simulink model "sampleModel1607_5"  (R2023a)
settings: Solver=VariableStepAuto  StartTime=0.0  StopTime=10.0  RelTol=1e-3
libraries: hdlsllib x2, simulink x1
settings Model: Creator=user1  LastModifiedBy=user1

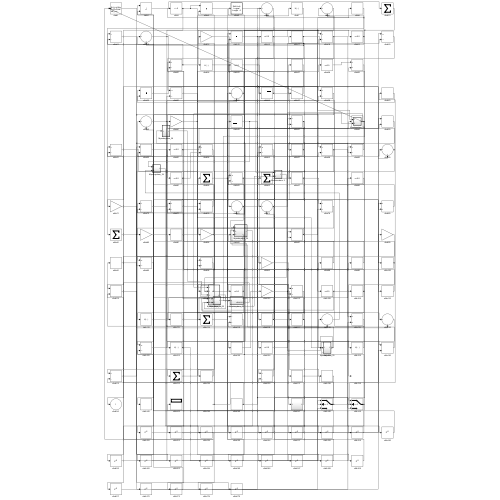
[thumbnail: Simulink's stored preview of the top-level diagram]
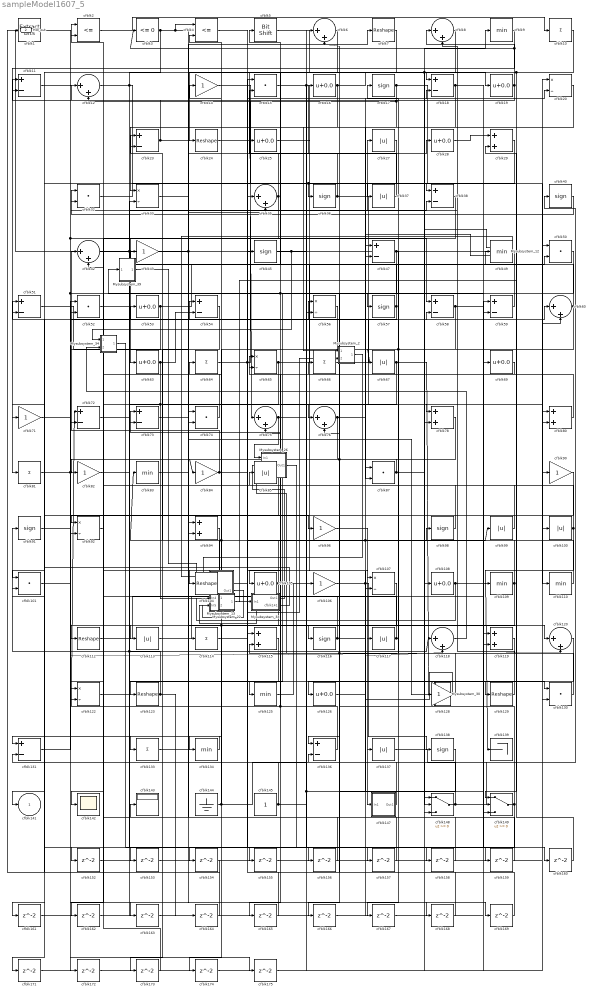
== system sampleModel1607_5 ==
  Mysubsystem_12 : Subsystem  TreatAsAtomicUnit=on  RTWFcnName=Mysubsystem_12
      settings: RTWFcnNameOpts=User specified  RTWFileNameOpts=Use function name
  Mysubsystem_13 : Subsystem  TreatAsAtomicUnit=on  RTWFcnName=Mysubsystem_13
      settings: RTWFcnNameOpts=User specified  RTWFileNameOpts=Use function name
  Mysubsystem_2 : Subsystem  TreatAsAtomicUnit=on  RTWFcnName=Mysubsystem_2
      settings: RTWFcnNameOpts=User specified  RTWFileNameOpts=Use function name
  Mysubsystem_22 : Subsystem  TreatAsAtomicUnit=on  RTWFcnName=Mysubsystem_22
      settings: RTWFcnNameOpts=User specified  RTWFileNameOpts=Use function name
  Mysubsystem_26 : Subsystem  TreatAsAtomicUnit=on  RTWFcnName=Mysubsystem_26
      settings: RTWFcnNameOpts=User specified  RTWFileNameOpts=Use function name
  Mysubsystem_30 : Subsystem  TreatAsAtomicUnit=on  RTWFcnName=Mysubsystem_30
      settings: RTWFcnNameOpts=User specified  RTWFileNameOpts=Use function name
  Mysubsystem_33 : Subsystem  TreatAsAtomicUnit=on  RTWFcnName=Mysubsystem_33
      settings: RTWFcnNameOpts=User specified  RTWFileNameOpts=Use function name
  Mysubsystem_34 : Subsystem  TreatAsAtomicUnit=on  RTWFcnName=Mysubsystem_34
      settings: RTWFcnNameOpts=User specified  RTWFileNameOpts=Use function name
  Mysubsystem_39 : Subsystem  TreatAsAtomicUnit=on  RTWFcnName=Mysubsystem_39
      settings: RTWFcnNameOpts=User specified  RTWFileNameOpts=Use function name
  cfblk1 : simulink/Logic and Bit Operations/Extract Bits  bitsToExtract=Upper half  numBits=8  bitIdxRange=[0 7]  outScalingMode=Preserve fixed-point scaling
      settings: LibrarySourceBlock=|
      | hdlsllib/Logic and Bit
      | Operations/Extract Bits
  cfblk{10,64,66,81,114,133} (6 alike) : Sum  Inputs=+  OutDataTypeStr=uint8
  cfblk{27,37,67,85,99..100,113,117,137} (9 alike) : Abs  OutDataTypeStr=uint8  SaturateOnIntegerOverflow=off
  cfblk{15,32,50,52,74,87,101,130} (8 alike) : DotProduct  OutDataTypeStr=uint8
  cfblk{7,24,104,112,123,129} (6 alike) : Reshape
  cfblk{16,19,25,28,53,63,69,105,108,126} (10 alike) : Bias  Bias=0.0  SaturateOnIntegerOverflow=off
  cfblk{14,43,71,82,84,90,96,106,128} (9 alike) : Gain  OutDataTypeStr=uint8
  cfblk{20,33,56,65,92,107,122} (7 alike) : Product  Inputs=*/  OutDataTypeStr=uint8  RndMeth=Zero  SaturateOnIntegerOverflow=on
  cfblk{9,49,83,109..110,125,134} (7 alike) : MinMax  OutDataTypeStr=uint8
  cfblk{11,18,23,38,47,51,54,58..59,72..73,131,136} (13 alike) : Sum  Inputs=+-  OutDataTypeStr=uint8
  cfblk{29,78,80,94,115,119} (6 alike) : Sum  OutDataTypeStr=uint8
  cfblk{17,36,40,45,57,91,98,116,138} (9 alike) : Signum
  cfblk{6,8,12,35,42,60,75..76,118,120} (10 alike) : Sum  Inputs=|++  OutDataTypeStr=uint8
  cfblk139 : Terminator
  cfblk142 : Scope
  cfblk143 : Display
  cfblk144 : Ground
  cfblk145 : Constant  OutDataTypeStr=uint8  SampleTime=-1
  cfblk147 : Subsystem
      settings: LibrarySourceBlock=|
      | hdlsllib/Ports &
      | Subsystems/Subsystem
  cfblk148 : Switch  OutDataTypeStr=uint8  SaturateOnIntegerOverflow=off  InputSameDT=off
  cfblk149 : Switch  OutDataTypeStr=uint8  SaturateOnIntegerOverflow=off  InputSameDT=off
  cfblk{152..169,171..175} (23 alike) : Delay  SampleTime=1
  cfblk2 : RelationalOperator  Operator=<=  OutDataTypeStr=boolean  InputSameDT=off
  cfblk3 : hdlsllib/Logic and Bit Operations/Compare To Zero  relop=<=  OutDataTypeStr=uint8
  cfblk4 : RelationalOperator  Operator=<=  OutDataTypeStr=boolean  InputSameDT=off
  cfblk5 : hdlsllib/Logic and Bit Operations/Bit Shift  mode=Shift Left Logical  N=0
  cfblk141 : Outport  OutDataTypeStr=uint8  VectorParamsAs1DForOutWhenUnconnected=off
  Hdl_out : Outport  Port=2  OutDataTypeStr=uint8
  wires:
  cfblk10/1 -> Mysubsystem_12/1(In1), cfblk75/1, cfblk149/1
  cfblk27/1 -> cfblk73/1
  cfblk9/1 -> cfblk81/1
  cfblk47/1 -> cfblk67/1, cfblk167/1, cfblk123/1
  cfblk64/1 -> cfblk27/1, cfblk107/1
  cfblk35/1 -> cfblk63/1, cfblk15/2
  cfblk6/1 -> Mysubsystem_39/1(In1), cfblk165/1
  cfblk75/1 -> Mysubsystem_26/1(In1), cfblk129/1
  cfblk84/1 -> cfblk42/1, cfblk18/2
  cfblk2/1 -> cfblk10/1
  cfblk136/1 -> cfblk72/1, cfblk85/1
  cfblk120/1 -> cfblk143/1
  cfblk78/1 -> cfblk84/1, cfblk116/1
  cfblk108/1 -> Mysubsystem_13/4(In4), cfblk139/1
  cfblk110/1 -> cfblk83/1, cfblk54/1
  cfblk24/1 -> cfblk100/1
  cfblk125/1 -> cfblk106/1
  cfblk32/1 -> cfblk38/1
  cfblk67/1 -> cfblk128/1, cfblk125/1
  cfblk15/1 -> cfblk147/1(In1), cfblk107/2
  cfblk99/1 -> cfblk65/1
  cfblk3/1 -> cfblk4/1, cfblk120/1, cfblk71/1
  cfblk60/1 -> cfblk126/1, cfblk23/1
  cfblk107/1 -> cfblk133/1, cfblk174/1
  cfblk65/1 -> cfblk49/1, cfblk113/1
  cfblk137/1 -> cfblk40/1
  cfblk149/1 -> cfblk66/1, cfblk171/1
  cfblk96/1 -> cfblk137/1
  cfblk106/1 -> cfblk138/1, cfblk118/2
  cfblk123/1 -> cfblk91/1, cfblk164/1
  cfblk36/1 -> cfblk110/1, cfblk25/1
  cfblk117/1 -> cfblk4/2, cfblk157/1
  cfblk130/1 -> cfblk17/1
  cfblk57/1 -> cfblk5/1, cfblk51/2
  cfblk109/1 -> cfblk43/1, cfblk162/1
  cfblk104/1 -> cfblk73/2, cfblk98/1
  cfblk82/1 -> cfblk56/1
  cfblk49/1 -> Mysubsystem_33/1(In1), cfblk117/1
  cfblk20/1 -> cfblk105/1
  cfblk98/1 -> cfblk2/1
  cfblk94/1 -> cfblk112/1
  cfblk8/1 -> cfblk24/1
  cfblk134/1 -> cfblk131/1
  cfblk129/1 -> cfblk32/1
  cfblk105/1 -> cfblk14/1, cfblk173/1
  cfblk119/1 -> cfblk115/2
  cfblk17/1 -> cfblk33/1, cfblk12/2, cfblk60/2
  cfblk37/1 -> cfblk16/1
  cfblk38/1 -> cfblk142/1
  cfblk7/1 -> cfblk75/2
  cfblk14/1 -> cfblk37/1
  cfblk126/1 -> cfblk99/1, cfblk20/2
  cfblk76/1 -> Mysubsystem_12/2(In2), cfblk94/2
  cfblk128/1 -> Mysubsystem_26/3(In3), cfblk6/2
  cfblk28/1 -> cfblk29/1
  cfblk42/1 -> cfblk38/2, cfblk130/1
  cfblk116/1 -> cfblk2/2, cfblk149/3
  cfblk18/1 -> cfblk119/1, cfblk87/2
  cfblk19/1 -> cfblk8/1, cfblk3/1, cfblk11/2
  cfblk63/1 -> Mysubsystem_22/1(In1), cfblk92/1, cfblk54/2
  cfblk5/1 -> cfblk148/2
  cfblk59/1 -> cfblk57/1
  cfblk80/1 -> cfblk8/2
  cfblk100/1 -> cfblk109/1, cfblk23/2
  cfblk16/1 -> Mysubsystem_2/1(In1), cfblk19/1
  cfblk72/1 -> cfblk78/1
  cfblk56/1 -> cfblk104/1
  cfblk33/1 -> cfblk35/2
  cfblk25/1 -> cfblk58/1
  cfblk144/1 -> cfblk64/1, cfblk6/1
  cfblk147/1(Out1) -> cfblk51/1
  cfblk45/1 -> Mysubsystem_34/1(In1), cfblk159/1
  cfblk131/1 -> cfblk52/1
  cfblk90/1 -> cfblk122/1
  cfblk51/1 -> cfblk74/2
  cfblk87/1 -> cfblk82/1, cfblk9/1
  cfblk122/1 -> cfblk50/2, cfblk118/1
  cfblk1/1 -> cfblk59/2, cfblk120/2
  cfblk12/1 -> cfblk108/1, cfblk18/1, cfblk154/1
  cfblk113/1 -> cfblk45/1
  cfblk69/1 -> cfblk65/2
  cfblk85/1 -> cfblk101/1
  cfblk74/1 -> cfblk12/1
  cfblk58/1 -> cfblk76/1, cfblk160/1
  cfblk53/1 -> cfblk20/1, cfblk92/2
  cfblk50/1 -> cfblk136/1
  cfblk23/1 -> cfblk11/1, cfblk169/1
  cfblk11/1 -> cfblk47/2, cfblk168/1
  cfblk112/1 -> cfblk69/1
  cfblk83/1 -> cfblk7/1
  cfblk115/1 -> cfblk134/1
  cfblk66/1 -> cfblk58/2
  cfblk81/1 -> cfblk53/1, cfblk96/1
  cfblk52/1 -> cfblk80/2
  cfblk148/1 -> cfblk90/1, cfblk52/2
  cfblk133/1 -> cfblk94/1
  cfblk29/1 -> cfblk36/1, cfblk161/1
  cfblk43/1 -> cfblk114/1, cfblk28/1
  cfblk40/1 -> cfblk32/2
  cfblk145/1 -> cfblk60/1, cfblk149/2, cfblk101/2
  cfblk92/1 -> cfblk152/1
  cfblk152/1 -> cfblk35/1
  cfblk54/1 -> cfblk153/1
  cfblk153/1 -> cfblk50/1
  cfblk154/1 -> cfblk1/1
  cfblk155/1 -> cfblk80/1
  cfblk4/1 -> cfblk156/1
  cfblk156/1 -> cfblk42/2
  cfblk157/1 -> cfblk122/2
  cfblk158/1 -> cfblk74/1
  cfblk159/1 -> cfblk76/2
  cfblk160/1 -> cfblk29/2
  cfblk161/1 -> cfblk78/2
  cfblk162/1 -> cfblk33/2
  cfblk91/1 -> cfblk163/1
  cfblk163/1 -> cfblk119/2
  cfblk164/1 -> cfblk131/2
  cfblk165/1 -> cfblk115/1
  cfblk138/1 -> cfblk166/1
  cfblk166/1 -> cfblk47/1
  cfblk167/1 -> cfblk148/3
  cfblk168/1 -> cfblk15/1
  cfblk169/1 -> cfblk136/2
  cfblk171/1 -> cfblk56/2
  cfblk71/1 -> cfblk172/1
  cfblk172/1 -> cfblk59/1
  cfblk173/1 -> cfblk72/2
  cfblk174/1 -> cfblk130/2
  cfblk101/1 -> cfblk175/1
  cfblk175/1 -> cfblk148/1
  cfblk114/1 -> Mysubsystem_2/2(In2)
  Mysubsystem_12/1(Out1) -> Mysubsystem_13/1(In1), Hdl_out/1
  Mysubsystem_2/1(Out1) -> Mysubsystem_13/2(In2)
  Mysubsystem_13/1(Out1) -> Mysubsystem_22/2(In2)
  Mysubsystem_22/1(Out1) -> Mysubsystem_13/5(In5)
  Mysubsystem_26/1(Out1) -> cfblk155/1
  cfblk73/1 -> Mysubsystem_30/1(In1)
  Mysubsystem_30/1(Out1) -> cfblk87/1
  Mysubsystem_33/1(Out1) -> Mysubsystem_26/2(In2)
  Mysubsystem_33/2(cfblk141) -> cfblk141/1
  cfblk118/1 -> Mysubsystem_34/2(In2)
  Mysubsystem_34/1(Out1) -> cfblk158/1
  Mysubsystem_39/1(Out1) -> Mysubsystem_13/3(In3)

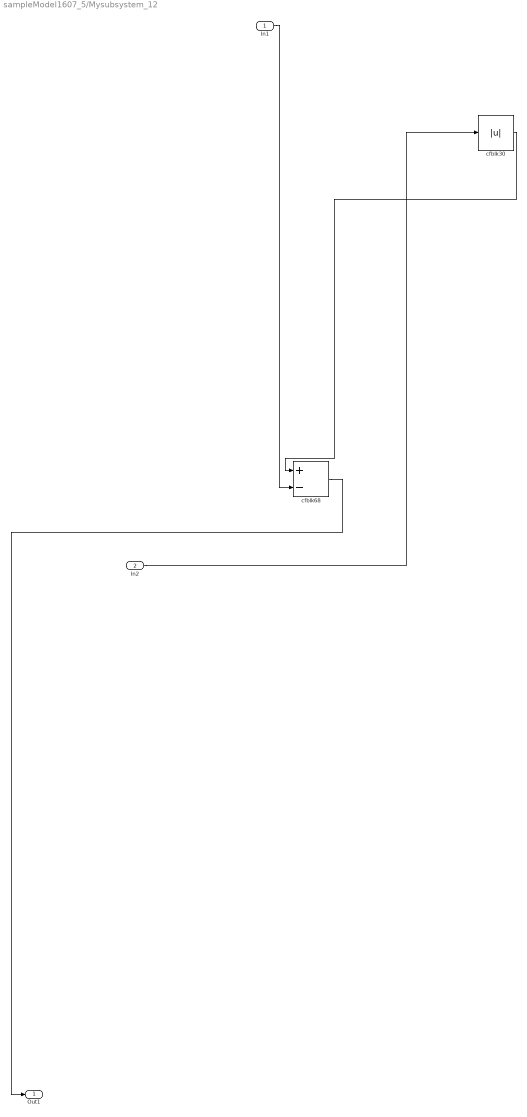
== system sampleModel1607_5/Mysubsystem_12 ==
  In1 : Inport
  In2 : Inport  Port=2
  cfblk30 : Abs  SaturateOnIntegerOverflow=off
  cfblk68 : Sum  Inputs=+-
  Out1 : Outport
  wires:
  cfblk30/1 -> cfblk68/1
  In1/1 -> cfblk68/2
  In2/1 -> cfblk30/1
  cfblk68/1 -> Out1/1

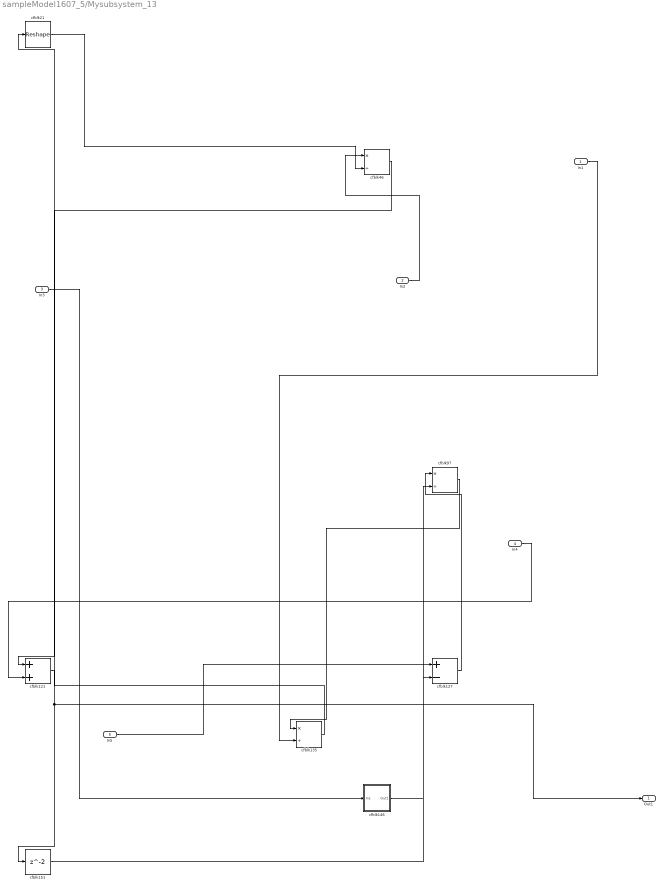
== system sampleModel1607_5/Mysubsystem_13 ==
  In1 : Inport
  In2 : Inport  Port=2
  In3 : Inport  Port=3
  In4 : Inport  Port=4
  In5 : Inport  Port=5
  cfblk121 : Sum
  cfblk127 : Sum  Inputs=+-
  cfblk135 : Product  Inputs=*/  RndMeth=Zero  SaturateOnIntegerOverflow=on
  cfblk146 : Subsystem
      settings: LibrarySourceBlock=|
      | hdlsllib/Ports &
      | Subsystems/Subsystem
  cfblk151 : Delay  SampleTime=1
  cfblk21 : Reshape
  cfblk46 : Product  Inputs=*/  RndMeth=Zero  SaturateOnIntegerOverflow=on
  cfblk97 : Product  Inputs=*/  RndMeth=Zero  SaturateOnIntegerOverflow=on
  Out1 : Outport
  wires:
  cfblk46/1 -> cfblk121/1
  cfblk135/1 -> cfblk21/1
  cfblk97/1 -> cfblk135/1
  cfblk146/1(Out1) -> cfblk97/2
  cfblk151/1 -> cfblk127/2
  cfblk121/1 -> Out1/1, cfblk151/1
  cfblk127/1 -> cfblk97/1
  cfblk21/1 -> cfblk46/2
  In5/1 -> cfblk127/1
  In3/1 -> cfblk146/1(In1)
  In2/1 -> cfblk46/1
  In1/1 -> cfblk135/2
  In4/1 -> cfblk121/2

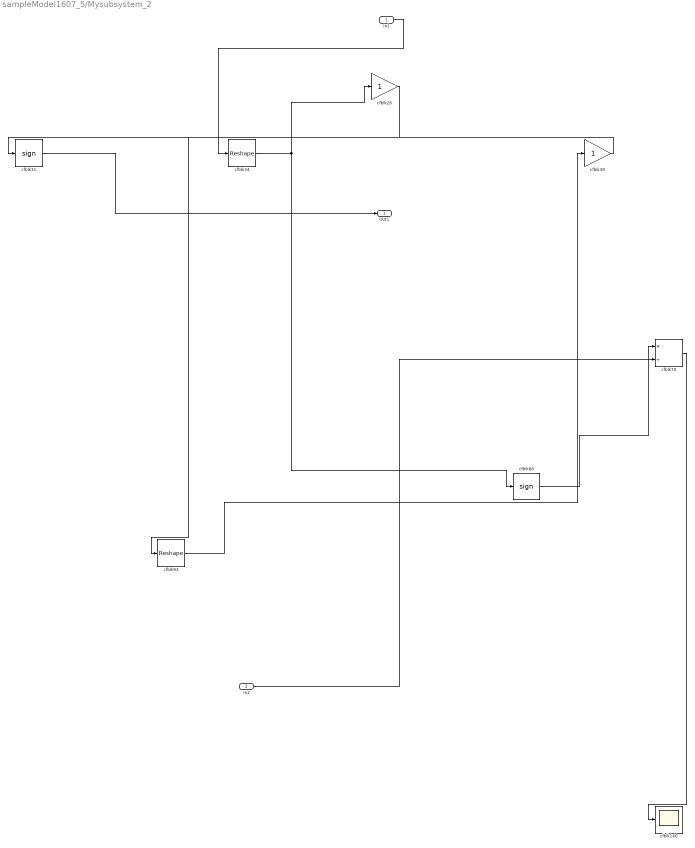
== system sampleModel1607_5/Mysubsystem_2 ==
  In1 : Inport
  In2 : Inport  Port=2
  cfblk140 : Scope
  cfblk26 : Gain
  cfblk31 : Signum
  cfblk34 : Reshape
  cfblk39 : Gain
  cfblk70 : Product  Inputs=*/  RndMeth=Zero  SaturateOnIntegerOverflow=on
  cfblk88 : Signum
  cfblk93 : Reshape
  Out1 : Outport
  wires:
  cfblk31/1 -> Out1/1
  cfblk70/1 -> cfblk140/1
  cfblk26/1 -> cfblk93/1
  cfblk39/1 -> cfblk31/1
  cfblk88/1 -> cfblk70/1
  In1/1 -> cfblk34/1
  cfblk34/1 -> cfblk88/1, cfblk26/1
  cfblk93/1 -> cfblk39/1
  In2/1 -> cfblk70/2

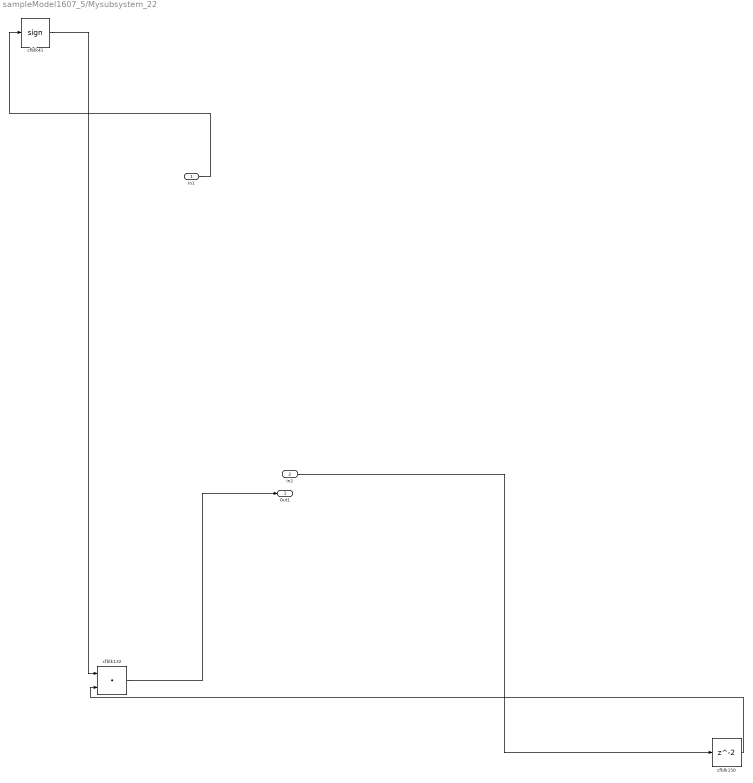
== system sampleModel1607_5/Mysubsystem_22 ==
  In1 : Inport
  In2 : Inport  Port=2
  cfblk132 : DotProduct  OutDataTypeStr=Inherit: Inherit via internal rule
  cfblk150 : Delay  SampleTime=1
  cfblk41 : Signum
  Out1 : Outport
  wires:
  In2/1 -> cfblk150/1
  cfblk150/1 -> cfblk132/2
  cfblk41/1 -> cfblk132/1
  In1/1 -> cfblk41/1
  cfblk132/1 -> Out1/1

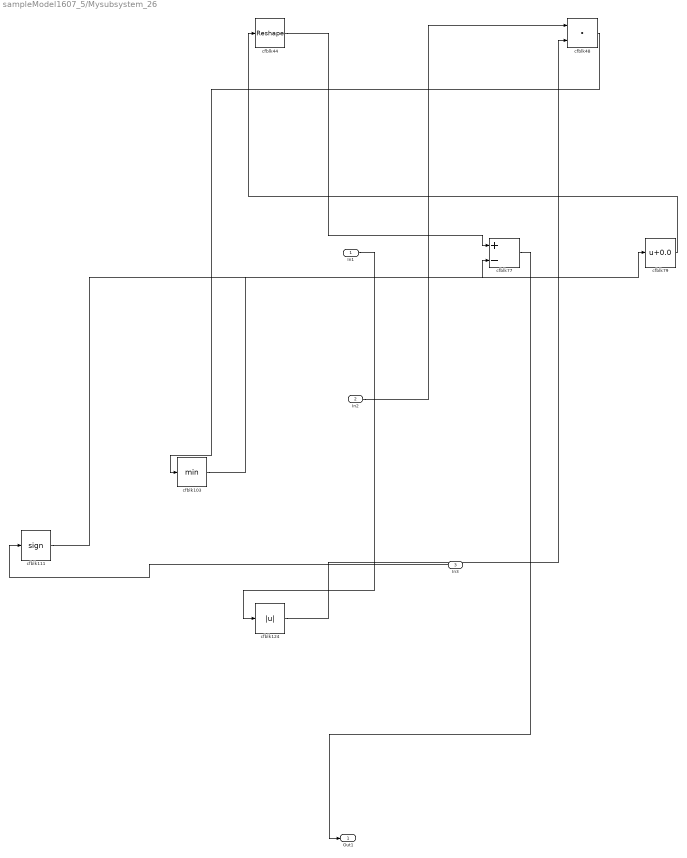
== system sampleModel1607_5/Mysubsystem_26 ==
  In1 : Inport
  In2 : Inport  Port=2
  In3 : Inport  Port=3
  cfblk103 : MinMax
  cfblk111 : Signum
  cfblk124 : Abs  SaturateOnIntegerOverflow=off
  cfblk44 : Reshape
  cfblk48 : DotProduct  OutDataTypeStr=Inherit: Inherit via internal rule
  cfblk77 : Sum  Inputs=+-
  cfblk79 : Bias  Bias=0.0  SaturateOnIntegerOverflow=off
  Out1 : Outport
  wires:
  cfblk79/1 -> cfblk44/1
  cfblk77/1 -> Out1/1
  cfblk103/1 -> cfblk77/2
  cfblk124/1 -> cfblk48/2
  cfblk48/1 -> cfblk103/1
  cfblk111/1 -> cfblk79/1
  cfblk44/1 -> cfblk77/1
  In1/1 -> cfblk124/1
  In2/1 -> cfblk48/1
  In3/1 -> cfblk111/1

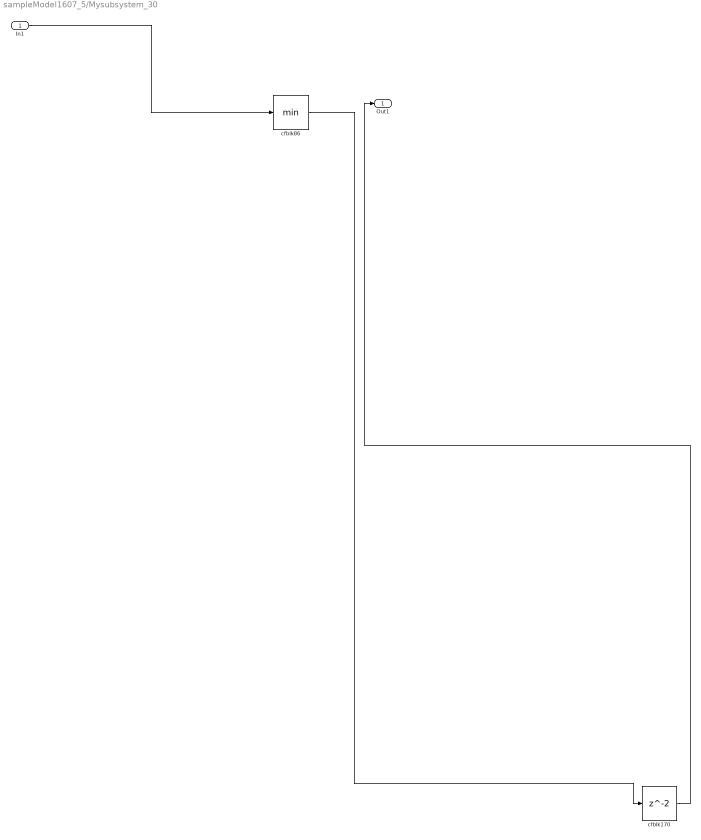
== system sampleModel1607_5/Mysubsystem_30 ==
  In1 : Inport
  cfblk170 : Delay  SampleTime=1
  cfblk86 : MinMax
  Out1 : Outport
  wires:
  In1/1 -> cfblk86/1
  cfblk86/1 -> cfblk170/1
  cfblk170/1 -> Out1/1

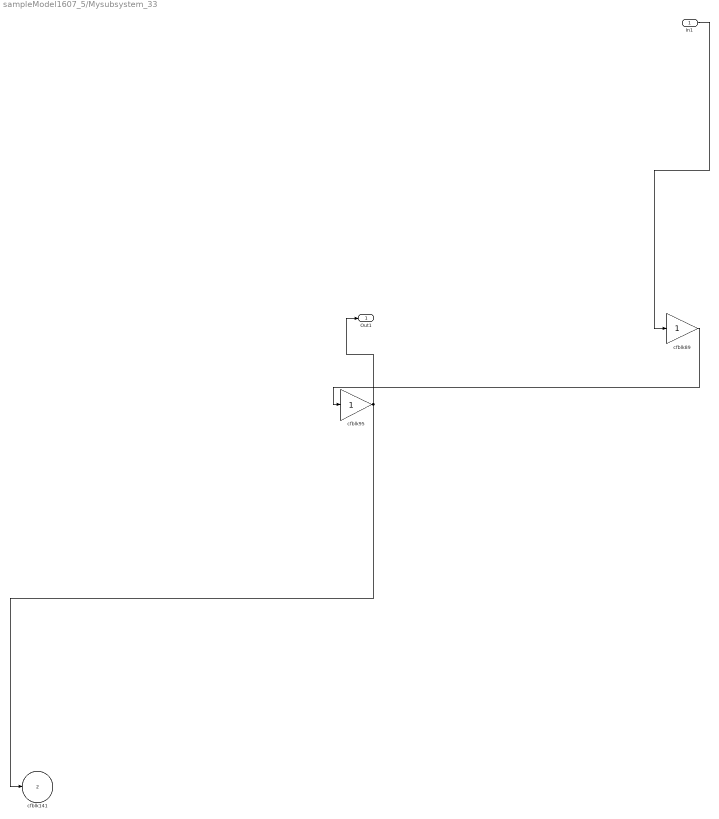
== system sampleModel1607_5/Mysubsystem_33 ==
  In1 : Inport
  cfblk89 : Gain
  cfblk95 : Gain
  Out1 : Outport
  cfblk141 : Outport  Port=2  VectorParamsAs1DForOutWhenUnconnected=off
  wires:
  cfblk95/1 -> cfblk141/1, Out1/1
  cfblk89/1 -> cfblk95/1
  In1/1 -> cfblk89/1

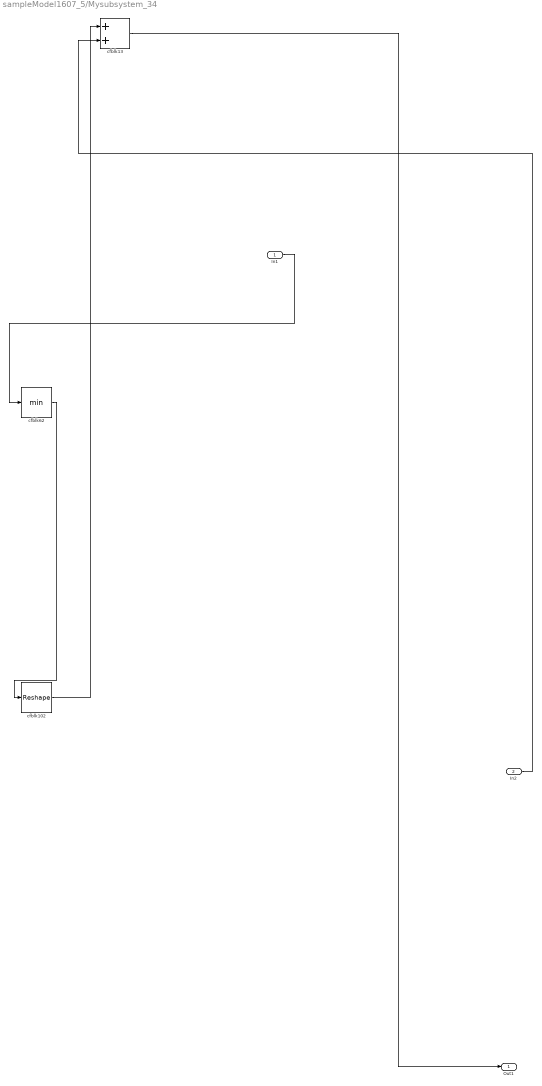
== system sampleModel1607_5/Mysubsystem_34 ==
  In1 : Inport
  In2 : Inport  Port=2
  cfblk102 : Reshape
  cfblk13 : Sum
  cfblk62 : MinMax
  Out1 : Outport
  wires:
  cfblk13/1 -> Out1/1
  cfblk102/1 -> cfblk13/1
  cfblk62/1 -> cfblk102/1
  In2/1 -> cfblk13/2
  In1/1 -> cfblk62/1

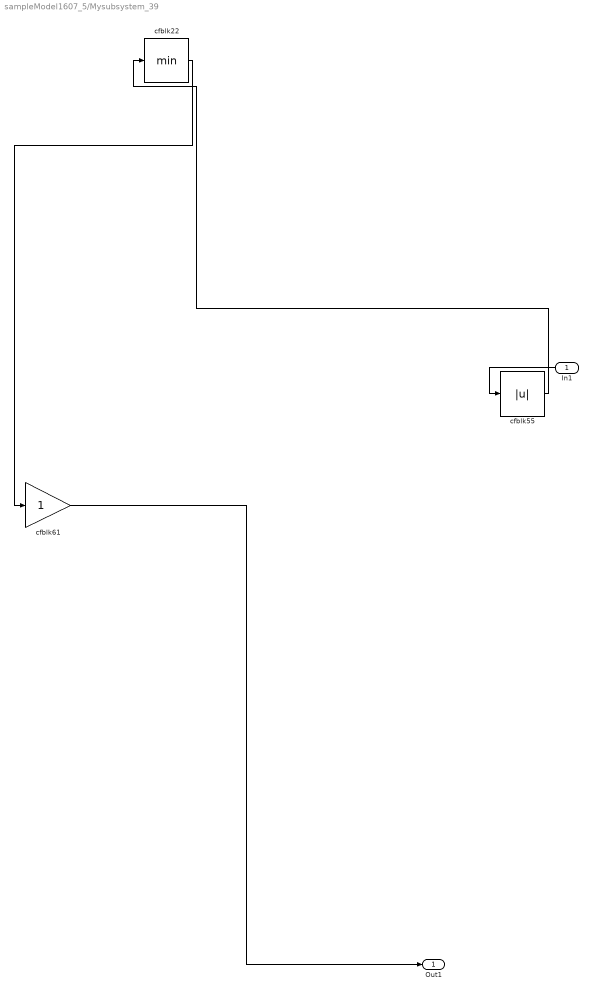
== system sampleModel1607_5/Mysubsystem_39 ==
  In1 : Inport
  cfblk22 : MinMax
  cfblk55 : Abs  SaturateOnIntegerOverflow=off
  cfblk61 : Gain
  Out1 : Outport
  wires:
  cfblk55/1 -> cfblk22/1
  In1/1 -> cfblk55/1
  cfblk22/1 -> cfblk61/1
  cfblk61/1 -> Out1/1

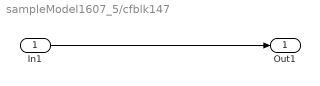
== system sampleModel1607_5/cfblk147 ==
  In1 : Inport
  Out1 : Outport
  wires:
  In1/1 -> Out1/1

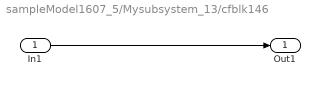
== system sampleModel1607_5/Mysubsystem_13/cfblk146 ==
  In1 : Inport
  Out1 : Outport
  wires:
  In1/1 -> Out1/1
